simulink model "sysgenStreamedFFT"  (Simulink 7.4)
settings: Solver=VariableStepDiscrete  StartTime=0.0  StopTime=3000  RelTol=1e-3
values from neighbouring files (symbols this model uses):
  blue = blue(1:(min_x*min_y))    [makematrix.m]    (also in rgb.mat = [0 0 0 255 255 255 255 255 255 0 0 0 ... (256 elements, 256x)
  c = c(:)    [cellpipe_r13.m]    (also in cordic_sincos_script.m = xSignal; get_pipestr_r13.m = cellpipe_r13(pipestr))
  comp = [zeros(70,2) [zeros(2,66); comp; zeros(2,66)] zeros(70,2)]    [sysgenDWT_StopFcn.m]
undefined symbols (not defined in the file or in its folder): gcbh, xlBlockLoadCallback, xlipgetpartsetting
libraries: xbsIndex_r4 x117, dspxfrm3 x2, xbsCopyrightNotice_r4 x1
(part 3 of 3)

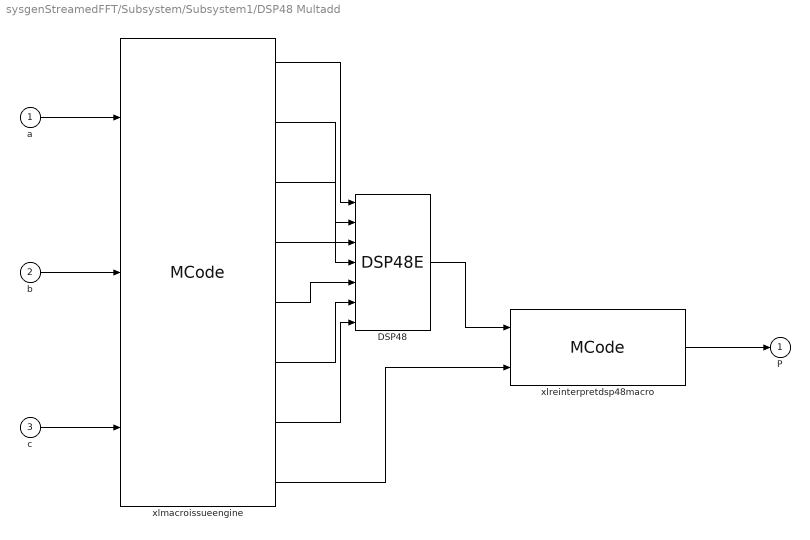
== system sysgenStreamedFFT/Subsystem/Subsystem1/DSP48 Multadd ==
  a : Inport  OutDataType=sfix(16)  OutScaling=2^0
  b : Inport  Port=2  OutDataType=sfix(16)  OutScaling=2^0
  c : Inport  Port=3  OutDataType=sfix(16)  OutScaling=2^0
  DSP48 : xbsIndex_r4/DSP48E  use_a=Direct from A Port  use_b=Direct from B Port  pattern_from_creg=off  pattern='000000000000'  mask_from_creg=off  pattern_mask='000000000000'  reset_preg=off  sel_rounding_mask=Select mask  use_op=off  use_creg=on  rst_all=off  en_all=off  use_pcin=off  use_carrycascin=off  use_multsignin=off  use_carryout=off  use_patterndetect=off  use_patternbdetect=off  use_overflow=off  use_underflow=off  use_acout=off  use_bcout=off  use_pcout=off  use_multsignout=off  use_carrycascout=off  pipeline_a=1  pipeline_b=1  pipeline_acout=1  pipeline_bcout=1  pipeline_c=on  pipeline_p=on  pipeline_mult=on  pipeline_opmode=on  pipeline_alumode=on  pipeline_carryin=on  pipeline_carryinsel=on  rst_a=off  rst_b=off  rst_c=off  rst_mult=off  rst_p=off  rst_carry_in=off  rst_alumode=off  rst_ctrl=off  en_a1=off  en_a2=off  en_b1=off  en_b2=off  en_c=off  en_mult=off  en_p=off  en_carry_in=off  en_alumode=off  en_multcarryin=off  en_ctrl=off  use_synth_model=off  addsub_mode=ONE48  xl_useadderonly=off  block_type=dsp48e
      settings: block_version=11.3
  xlmacroissueengine : xbsIndex_r4/MCode  mfname=xlissue_engine_v5  explicit_period=off  period=inf  dbl_ovrd=off  enable_stdout=off  enable_debug=off  suppress_output=on  defparams={'id_a1', 0,'id_a2', 0,'id_a3', 0,'id_a4', 0,'id_a5', 0,'id_a6', 0,'id_a7', 0,'id_b1', 0,'id_b2', 0,'id_b3', 0,'id_b4', 0,'id_b5', 0,'id_b6', 0,'id_b7', 0,'id_c1', 0,'id_c2', 0,'id_c3', 0,'id_c4', 0,'id_c5', 0,'id_c6', 0,'id_c7', 0,'op_const0',53,'op_const1', 0,'op_const2', 0,'op_const3', 0,'op_const4', 0,'op_const5', 0,'op_const6', 0,'op_const7', 0,'alumode_const0',0,'alumode_const1', 0,'alumode_const2', 0,'alumode_const3', 0,'alumode_const4', 0,'alumode_const5', 0,'alumode_const6', 0,'alumode_const7', 0,'carry_in_sel0',0,'carry_in_sel1', 0,'carry_in_sel2', 0,'carry_in_sel3', 0,'carry_in_sel4', 0,'carry_in_sel5', 0,'carry_in_sel6', 0,'carry_in_sel7', 0,'external_cin0', 0,'external_cin1', 0,'external_cin2', 0,'external_cin3', 0,'external_cin4', 0,'external_cin5', 0,'external_cin6', 0,'external_cin7', 0,'reg_a',0,'reg_b',0,'reg_c',0,'reg_op',0,'mode0', 1,'mode1', 0,'mode2', 0,'mode3', 0,'mode4', 0,'mode5', 0,'mode6', 0,'mode7', 0,'ce_all',true,'use_ce_all',false,'sel',0,'rst_all',false,'use_rst_all',false,'cinused',false,'ninstr',1}  hide_port_list={}  block_type=mcode
      settings: xl_area=[0, 0, 0, 0, 0, 0, 0]  block_version=9.1
  xlreinterpretdsp48macro : xbsIndex_r4/MCode  mfname=xlreinterpretdsp48macro  explicit_period=off  period=1  dbl_ovrd=off  enable_stdout=off  enable_debug=off  suppress_output=off  defparams={'full',precision,'n_bits',n_bits,'bin_pt',bin_pt,'arith_type',arith_type}  hide_port_list={}  block_type=mcode
      settings: xl_area=[0, 0, 0, 0, 0, 0, 0]  block_version=9.1
  P : Outport  OutDataType=sfix(16)  OutScaling=2^0
  wires:
  xlreinterpretdsp48macro/1 -> P/1
  DSP48/1 -> xlreinterpretdsp48macro/1
  xlmacroissueengine/8 -> xlreinterpretdsp48macro/2
  xlmacroissueengine/7 -> DSP48/7
  xlmacroissueengine/6 -> DSP48/6
  xlmacroissueengine/5 -> DSP48/5
  xlmacroissueengine/4 -> DSP48/4
  xlmacroissueengine/3 -> DSP48/3
  xlmacroissueengine/2 -> DSP48/2
  xlmacroissueengine/1 -> DSP48/1
  c/1 -> xlmacroissueengine/3
  b/1 -> xlmacroissueengine/2
  a/1 -> xlmacroissueengine/1
